simulink model "EddyBrakeDynamicsA34"  (Simulink 8.5)
settings: Solver=ode45  StartTime=0.0  StopTime=10.0  RelTol=1e-3
settings Model: Creator=MrPiccolo  LastModifiedBy=MrPiccolo
settings DataIOCC: SignalLoggingSaveFormat=Dataset
settings OptimizationCC: ExpressionDepthLimit=128
settings DebuggingCC: UnderspecifiedInitializationDetection=Simplified  MergeDetectMultiDrivingBlocksExec=error  FcnCallInpInsideContextMsg=EnableAllAsError  StateNameClashWarn=none
settings GRTTargetCC: CombineOutputUpdateFcns=on  GRTInterface=off

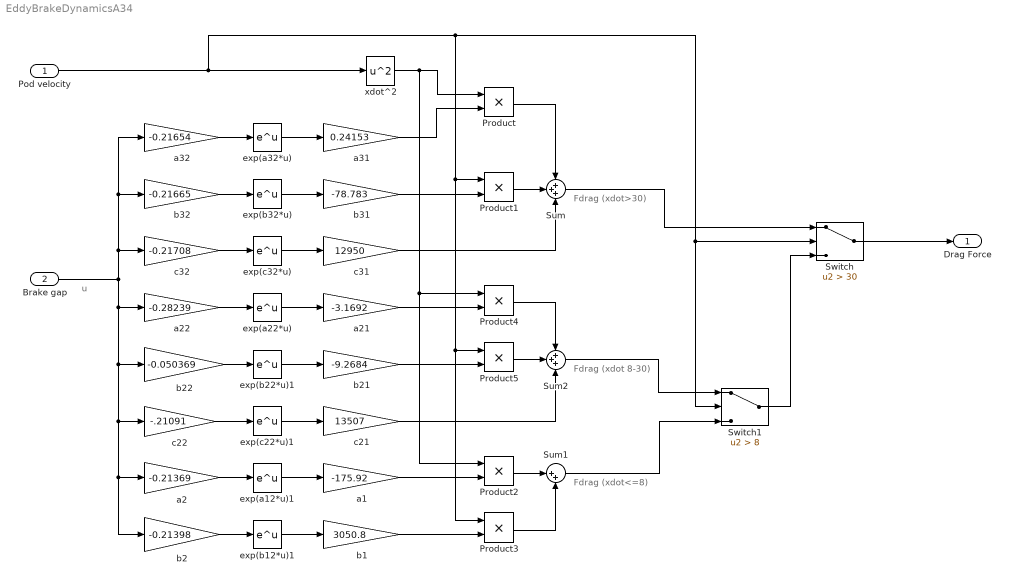
== system EddyBrakeDynamicsA34 ==
  note: Fdrag (xdot>30)
  note: u
  note: Fdrag (xdot<=8)
  note: Fdrag (xdot 8-30)
  Pod velocity : Inport
  Brake gap : Inport  Port=2
  Product{,1..5} (6 alike) : Product
  Sum : Sum  Inputs=+++
  Sum1 : Sum  Inputs=|++
  Sum2 : Sum  Inputs=+++
  Switch : Switch  Criteria=u2 > Threshold  Threshold=30
  Switch1 : Switch  Criteria=u2 > Threshold  Threshold=8
  a1 : Gain  Gain=-175.92
  a2 : Gain  Gain=-0.21369
  a21 : Gain  Gain=-3.1692
  a22 : Gain  Gain=-0.28239
  a31 : Gain  Gain=0.24153
  a32 : Gain  Gain=-0.21654
  b1 : Gain  Gain=3050.8
  b2 : Gain  Gain=-0.21398
  b21 : Gain  Gain=-9.2684
  b22 : Gain  Gain=-0.050369
  b31 : Gain  Gain=-78.783
  b32 : Gain  Gain=-0.21665
  "c21 " : Gain  Gain=13507
  c22 : Gain  Gain=-.21091
  c31 : Gain  Gain=12950
  c32 : Gain  Gain=-0.21708
  exp(a12*u)1 : Math  SaturateOnIntegerOverflow=on
  exp(a22*u) : Math  SaturateOnIntegerOverflow=on
  exp(a32*u) : Math  SaturateOnIntegerOverflow=on
  exp(b12*u)1 : Math  SaturateOnIntegerOverflow=on
  exp(b22*u)1 : Math  SaturateOnIntegerOverflow=on
  exp(b32*u) : Math  SaturateOnIntegerOverflow=on
  exp(c22*u)1 : Math  SaturateOnIntegerOverflow=on
  exp(c32*u) : Math  SaturateOnIntegerOverflow=on
  xdot^2 : Math  Operator=square  SaturateOnIntegerOverflow=on
  Drag Force : Outport
  wires:
  a32/1 -> exp(a32*u)/1
  Product/1 -> Sum/1
  exp(a32*u)/1 -> a31/1
  xdot^2/1 -> Product/1, Product2/1, Product4/1
  b32/1 -> exp(b32*u)/1
  Product1/1 -> Sum/2
  a22/1 -> exp(a22*u)/1
  a31/1 -> Product/2
  exp(a22*u)/1 -> a21/1
  Pod velocity/1 -> Switch/2, Switch1/2, Product3/1, Product5/1, Product1/1, xdot^2/1
  b31/1 -> Product1/2
  Sum/1 -> Switch/1
  Product3/1 -> Sum1/2
  Product2/1 -> Sum1/1
  a1/1 -> Product2/2
  b1/1 -> Product3/2
  Switch/1 -> Drag Force/1
  Switch1/1 -> Switch/3
  exp(b32*u)/1 -> b31/1
  Product4/1 -> Sum2/1
  a21/1 -> Product4/2
  b22/1 -> exp(b22*u)1/1
  exp(b22*u)1/1 -> b21/1
  b21/1 -> Product5/2
  Product5/1 -> Sum2/2
  a2/1 -> exp(a12*u)1/1
  exp(a12*u)1/1 -> a1/1
  b2/1 -> exp(b12*u)1/1
  exp(b12*u)1/1 -> b1/1
  Brake gap/1 -> b2/1, a2/1, c22/1, b22/1, a22/1, c32/1, a32/1, b32/1
  c32/1 -> exp(c32*u)/1
  exp(c32*u)/1 -> c31/1
  c31/1 -> Sum/3
  Sum1/1 -> Switch1/3
  c22/1 -> exp(c22*u)1/1
  exp(c22*u)1/1 -> "c21 "/1
  "c21 "/1 -> Sum2/3
  Sum2/1 -> Switch1/1
